simulink model "EXPERIMENTS"  (R2020a)
settings: Solver=FixedStepDiscrete  StartTime=0.0  StopTime=10.0  FixedStep=0.1  RelTol=1e-3  EnableMultiTasking=on
settings Model: Creator=hp-pc  LastModifiedBy=hp-pc
settings SolverCC: AutoInsertRateTranBlk=on
settings DataIOCC: LimitDataPoints=on
settings OptimizationCC: LifeSpan=inf
settings DebuggingCC: AllowSymbolicDim=off  SFUnexpectedBacktrackingDiag=warning  SFNoUnconditionalDefaultTransitionDiag=warning  SFExecutionAtInitializationDiag=none  ArithmeticOperatorsInVariantConditions=warning
settings SFSimCC: SimUseLocalCustomCode=off  CustomCodeUndefinedFunction=UseInterfaceOnly
settings RTWCC: RTWUseLocalCustomCode=off
settings CodeAppCC: StateflowObjectComments=on
settings GRTTargetCC: TargetLangStandard=C89/C90 (ANSI)
settings ConfigComp: CovMetricSettings=dw  CovHtmlReporting=on  CovSaveCumulativeToWorkspaceVar=on  CovSaveSingleToWorkspaceVar=on  CovShowResultsExplorer=off  CovExternalEMLEnable=off  CovSFcnEnable=off

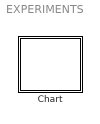
== system EXPERIMENTS ==
  Chart : Stateflow chart  TreatAsAtomicUnit=on

== stateflow chart EXPERIMENTS/Chart ==
  state C1
    C1_=1;
    w_NORTH_e_green = 1;w_SOUTH_e_green = 1;
    state w_NORTH_e [parallel]
      settings: executionOrder=1
      state Stop
        % Red light
        entry:
        red = 1;
        yellow = 0;
        green = 0;
      state PrepareToStop
        % Yellow light
        entry:
        red = 0;
        yellow = 1;
        green = 0;
      state Go
        % Green light
        entry:
        red = 0;
        yellow = 0;
        green = 1;
      (default) -> C1.w_NORTH_e.Stop
      C1.w_NORTH_e.Stop -> (junction 46)
      (junction 46) -> (junction 25) : after(3,sec)
      C1.w_NORTH_e.PrepareToStop -> C1.w_NORTH_e.Stop : after(3,sec)
      C1.w_NORTH_e.Go -> C1.w_NORTH_e.PrepareToStop : after(10,sec)
      (junction 25) -> C1.w_NORTH_e.Go
    state w_SOUTH_e [parallel]
      settings: executionOrder=2
      state Stop
        % Red light
        entry:
        red = 1;
        yellow = 0;
        green = 0;
      state PrepareToStop
        % Yellow light
        entry:
        red = 0;
        yellow = 1;
        green = 0;
      state Go
        % Green light
        entry:
        red = 0;
        yellow = 0;
        green = 1;
      (default) -> C1.w_SOUTH_e.Stop
      C1.w_SOUTH_e.Stop -> (junction 33)
      (junction 33) -> (junction 34) : after(3,sec)
      C1.w_SOUTH_e.PrepareToStop -> C1.w_SOUTH_e.Stop : after(3,sec)
      C1.w_SOUTH_e.Go -> C1.w_SOUTH_e.PrepareToStop : after(10,sec)
      (junction 34) -> C1.w_SOUTH_e.Go
  state C2
    C2_=1;
    s_WEST_n_green = 1;s_EAST_n_green = 1;
    state s_WEST_n [parallel]
      settings: executionOrder=2
      state Stop
        % Red light
        entry:
        red = 1;
        yellow = 0;
        green = 0;
      state PrepareToStop
        % Yellow light
        entry:
        red = 0;
        yellow = 1;
        green = 0;
      state Go
        % Green light
        entry:
        red = 0;
        yellow = 0;
        green = 1;
      (default) -> C2.s_WEST_n.Stop
      C2.s_WEST_n.Stop -> (junction 28)
      (junction 28) -> (junction 65) : after(3,sec)
      C2.s_WEST_n.PrepareToStop -> C2.s_WEST_n.Stop : after(3,sec)
      C2.s_WEST_n.Go -> C2.s_WEST_n.PrepareToStop : after(10,sec)
      (junction 65) -> C2.s_WEST_n.Go
    state s_EAST_n [parallel]
      settings: executionOrder=1
      state Stop
        % Red light
        entry:
        red = 1;
        yellow = 0;
        green = 0;
      state PrepareToStop
        % Yellow light
        entry:
        red = 0;
        yellow = 1;
        green = 0;
      state Go
        % Green light
        entry:
        red = 0;
        yellow = 0;
        green = 1;
      (default) -> C2.s_EAST_n.Stop
      C2.s_EAST_n.Stop -> (junction 51)
      (junction 51) -> (junction 52) : after(3,sec)
      C2.s_EAST_n.PrepareToStop -> C2.s_EAST_n.Stop : after(3,sec)
      C2.s_EAST_n.Go -> C2.s_EAST_n.PrepareToStop : after(10,sec)
      (junction 52) -> C2.s_EAST_n.Go
  note: %B7%North-SouthL  ALLrest R=1
      | %B2_=1;
      | %B1_GS = 1;B1_GL= 1;
      | %R=0;
      | %B1_=1;%parallel withB2
  state B2%North-SouthL  ALLrest R=1
    B2_=1;
    %B1_GS = 1;B1_GL= 1;
    %R=0;
    %B1_=1;%parallel withB2
    state B3%southL [parallel]
      B3_=1;
      B3_GS = 1;B3_GL= 1;
      B3_R=0;
      %B1_=0;B2_=0;
      REDrest=1;
      settings: executionOrder=1
    state B1%GL=GS=1,R=0,    ALLrest R=1 northL [parallel]
      B1_=1;
      B1_GS = 1;B1_GL= 1;
      B1_R=0;
      REDrest=1;
      settings: executionOrder=2
  state B3%southL
    B3_=1;
    B3_GS = 1;B3_GL= 1;
    B3_R=0;
    B1_=0;B2_=0;
    REDrest=1;
    B1_GS = 1;B1_GL= 0;
  state B1%GL=GS=1,R=0,    ALLrest R=1 northL
    B1_=1;
    B1_GS = 1;B1_GL= 1;
    B1_R=0;
    REDrest=1;
  state B5%West-EAST L
    B5_=1;
    %GS = 1;GL= 1;
    %R=0;
    B1_=0;B2_=0;B3_=0;
    B1_GS = 1;B1_GL= 0;
    %B4_=1;
    state B4%WestL [parallel]
      B4_=1;
      B4_GS = 1;B4_GL= 1;
      B4_R=0;
      B1_=0;B2_=0;B3_=0;
      REDrest=1;
      settings: executionOrder=1
    state B6%EASTL [parallel]
      B6_=1;
      B6_GS = 1;B6_GL= 1;
      B6_R=0;
      B1_=0;B2_=0;B3_=0;
      B4_=1;B5_=1;
      REDrest=1;
      settings: executionOrder=2
  state B4%WestL
    B4_=1;
    B4_GS = 1;B4_GL= 1;
    B4_R=0;
    B1_=0;B2_=0;B3_=0;
    REDrest=1;
    B1_GS = 0;B1_GL= 0;
    B3_GS = 0;B3_GL= 0;
  state B6%EASTL
    B6_=1;
    B6_GS = 1;B6_GL= 1;
    B6_R=0;
    B1_=0;B2_=0;B3_=0;
    B4_=0;B5_=0;
    REDrest=1;
    B3_GS = 0;B3_GL= 0;
    B1_GS = 0;B1_GL= 0;
  note: %B8%West-EAST L
      | %B5_=1;
      | %GS = 1;GL= 1;
      | %R=0;
      | %B1_=0;B2_=0;B3_=0;
      | %B4_=1;
      | ?
  (default) -> C1 [order 2]
  C1 -> C2 : after(90,sec)[(yellow == 1)]{w_NORTH_e_green = 0;w_SOUTH_e_green = 0;}
  C2 -> C1 : after(90,sec)[(yellow == 1)]{s_WEST_n_green = 0;s_EAST_n_green = 0;}
  B2%North-SouthL  ALLrest R=1 -> B3%southL : after(90,sec)
  (default) -> B1%GL=GS=1,R=0,    ALLrest R=1 northL [order 1]
  B3%southL -> B4%WestL : after(90,sec)
  B1%GL=GS=1,R=0,    ALLrest R=1 northL -> B2%North-SouthL  ALLrest R=1 : after(45,sec)
  B6%EASTL -> B1%GL=GS=1,R=0,    ALLrest R=1 northL : after(90,sec)
  B4%WestL -> B5%West-EAST L : after(45,sec)
  B5%West-EAST L -> B6%EASTL : after(90,sec)
